simulink subsystem "accelerometer"  (R2022b)
settings: Solver=VariableStepAuto  StartTime=0.0  StopTime=10.0  RelTol=1e-3
libraries: frdmk64flib x1, dspstat3 x1
settings Model: Creator=ethan  LastModifiedBy=ethan

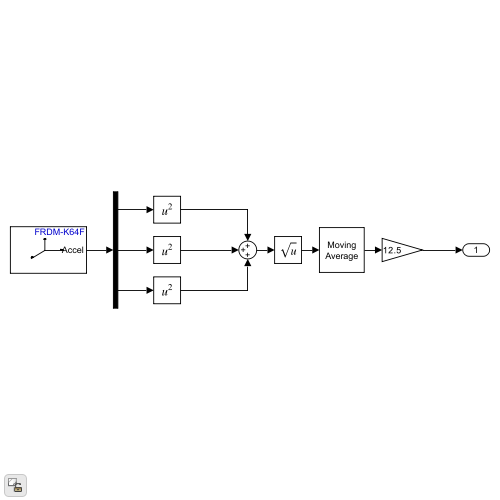
[thumbnail: Simulink's stored preview of the top-level diagram]
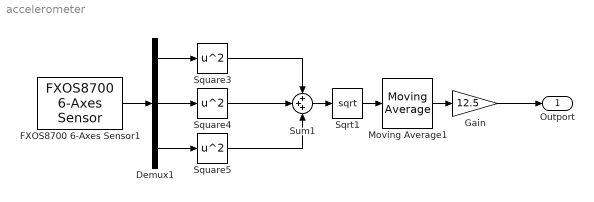
== system accelerometer ==
  Demux1 : Demux  Outputs=3
  FXOS8700 6-Axes Sensor1 : frdmk64flib/FXOS8700 6-Axes Sensor  Activesensor=Accelerometer only  ODR=800Hz  HybridODR=400Hz  Accelfullrange=-4g to +4g  SampleTime=-1
  Gain : Gain  Gain=12.5
  Moving Average1 : dspstat3/Moving Average  Method=Sliding window  ForgettingFactorPort=off  SpecifyWindowLength=on  WindowLength=4  OverlapLength=3  AllowArbitraryInputLength=off  ForgettingFactor=0.9  SimulateUsing=Code generation
  Sqrt1 : Sqrt
  Square3 : Math  Operator=square
  Square4 : Math  Operator=square
  Square5 : Math  Operator=square
  Sum1 : Sum  Inputs=+++
  Outport : Outport
  wires:
  Moving Average1/1 -> Gain/1
  Demux1/3 -> Square5/1
  Square3/1 -> Sum1/1
  Demux1/1 -> Square3/1
  FXOS8700 6-Axes Sensor1/1 -> Demux1/1
  Sum1/1 -> Sqrt1/1
  Demux1/2 -> Square4/1
  Square5/1 -> Sum1/3
  Sqrt1/1 -> Moving Average1/1
  Square4/1 -> Sum1/2
  Gain/1 -> Outport/1
